simulink model "Cooperative_Localization_05"  (R2016b)
settings: Solver=ode45  StartTime=0.0  StopTime=300  RelTol=1e-3  EnableMultiTasking=on
InitFcn:
  | Const_Coop_Local_05
undefined symbols (not defined in the file): alpha, AN, B, B_pseudo_inverse, BBT_inv, BN, D, Delta_form, Gama0, gamma0, gamma_0, gamma_1, H, K, k0_est, k1, k1_est, k2, KI, Ki_1, Ki_2, Ki_3, Ki_4, lambda, m_cont, Mb, Mu, n, N, n_cont, Observer_Gain, P_struct, Q, Q1, R, Rho1, Rho_0, rho_0, rho_1, t_cont, U_dot0_M
(part 3 of 3)

== matlab function Cooperative_Localization_05/Agent-3/observer-1 ==
  data: P_hat input; tau input; P0 input; P_rel_local input; P_rel0_local input; AN parameter; BN parameter; H parameter; DP_hat_local output; n parameter; N parameter; Num input; Mu parameter; Mb parameter; tau_i output; alpha parameter
function [DP_hat_local,tau_i] = fcn(P_hat,tau,P0,P_rel_local,P_rel0_local,AN,BN,H,n,N,Num,Mu,Mb,alpha)

P_hat_in = zeros(n,N);
P_rel_local_in = zeros(n,N);
tau_in = zeros(n,N);
for i=1:N
    P_hat_in(:,i) = P_hat((i-1)*n+1:(i*n),1); 
    P_rel_local_in(:,i) = P_rel_local((i-1)*n+1:(i*n),1); 
    tau_in(:,i) = tau((i-1)*n+1:(i*n),1);
end

e = BN(Num,Num)*(P_hat_in(:,Num) - (P0 + P_rel0_local));
Vec = zeros(n,1);
for i=1:N
    e = e + ( AN(Num,i)*(P_hat_in(:,Num) - (P_hat_in(:,i) + P_rel_local_in(:,i))) ); 
    Vec = Vec + ( H(Num,i)*tau_in(:,i) );    
end

SGN_vec = Vec./(abs(Vec)+alpha);
SGN = diag(SGN_vec);    

DP_hat_local = - ( Mu*e ) - ( SGN*Mb );
tau_i = e;

end

== matlab function Cooperative_Localization_05/Agent-4/Agent-4/MATLAB Function ==
  data: Vx input; out output; Vy input; Ax input; Ay input
function out = fcn(Vx,Vy,Ax,Ay)

DPx = Vx;
DPy = Vy;

DVx = Ax;
DVy = Ay;

out = [DPx;DPy;DVx;DVy];

end

== matlab function Cooperative_Localization_05/Agent-4/Relative positions-4/Differentiator_Scalar1/Sliding differentiator ==
  data: u output; u1 input; e_inp input; k1 parameter
function u = fcn(u1,e_inp,k1)

b=k1;

if e_inp>0
    ABS = e_inp;
else
    ABS = -e_inp;
end

SGN = e_inp/(ABS + 0.01);

u = u1 - b*(ABS^0.5)*SGN;

end

== matlab function Cooperative_Localization_05/Agent-4/Relative positions-4/Differentiator_Scalar1/Sliding differentiator1 ==
  data: Du1 output; e_inp input; k2 parameter
function Du1 = fcn(e_inp,k2)

a=k2;

if e_inp>0
    ABS = e_inp;
else
    ABS = -e_inp;
end
SGN = e_inp/(ABS + 0.01);

Du1 = - a*SGN;

end

== matlab function Cooperative_Localization_05/Agent-4/Relative positions-4/Differentiator_Scalar2/Sliding differentiator ==
  data: u output; u1 input; e_inp input; k1 parameter
function u = fcn(u1,e_inp,k1)

b=k1;

if e_inp>0
    ABS = e_inp;
else
    ABS = -e_inp;
end

SGN = e_inp/(ABS + 0.01);

u = u1 - b*(ABS^0.5)*SGN;

end

== matlab function Cooperative_Localization_05/Agent-4/Relative positions-4/Differentiator_Scalar2/Sliding differentiator1 ==
  data: Du1 output; e_inp input; k2 parameter
function Du1 = fcn(e_inp,k2)

a=k2;

if e_inp>0
    ABS = e_inp;
else
    ABS = -e_inp;
end
SGN = e_inp/(ABS + 0.01);

Du1 = - a*SGN;

end

== matlab function Cooperative_Localization_05/Agent-4/Relative positions-4/Differentiator_Scalar3/Sliding differentiator ==
  data: u output; u1 input; e_inp input; k1 parameter
function u = fcn(u1,e_inp,k1)

b=k1;

if e_inp>0
    ABS = e_inp;
else
    ABS = -e_inp;
end

SGN = e_inp/(ABS + 0.01);

u = u1 - b*(ABS^0.5)*SGN;

end

== matlab function Cooperative_Localization_05/Agent-4/Relative positions-4/Differentiator_Scalar3/Sliding differentiator1 ==
  data: Du1 output; e_inp input; k2 parameter
function Du1 = fcn(e_inp,k2)

a=k2;

if e_inp>0
    ABS = e_inp;
else
    ABS = -e_inp;
end
SGN = e_inp/(ABS + 0.01);

Du1 = - a*SGN;

end

== matlab function Cooperative_Localization_05/Agent-4/Relative positions-4/Differentiator_Scalar4/Sliding differentiator ==
  data: u output; u1 input; e_inp input; k1 parameter
function u = fcn(u1,e_inp,k1)

b=k1;

if e_inp>0
    ABS = e_inp;
else
    ABS = -e_inp;
end

SGN = e_inp/(ABS + 0.01);

u = u1 - b*(ABS^0.5)*SGN;

end

== matlab function Cooperative_Localization_05/Agent-4/Relative positions-4/Differentiator_Scalar4/Sliding differentiator1 ==
  data: Du1 output; e_inp input; k2 parameter
function Du1 = fcn(e_inp,k2)

a=k2;

if e_inp>0
    ABS = e_inp;
else
    ABS = -e_inp;
end
SGN = e_inp/(ABS + 0.01);

Du1 = - a*SGN;

end

== matlab function Cooperative_Localization_05/Agent-4/Relative positions-4/Relative estimation1 ==
  data: V_rel input; d input; DP_est output; Dot_d input; P_est input; k0_est parameter; k1_est parameter
function DP_est = fcn(V_rel,d,Dot_d,P_est,k0_est,k1_est)

D = d*Dot_d;
e = (d^2) - (P_est'*P_est);
g = P_est'*V_rel;
DP_est = zeros(2,1);

if (V_rel'*V_rel) > 0
    beta = (k1_est*D + k0_est*e) / (k1_est*g+0.001);
    DP_est = beta * V_rel;
end

end

== matlab function Cooperative_Localization_05/Agent-4/Relative positions-4/Relative estimation2 ==
  data: V_rel input; d input; DP_est output; Dot_d input; P_est input; k0_est parameter; k1_est parameter
function DP_est = fcn(V_rel,d,Dot_d,P_est,k0_est,k1_est)

D = d*Dot_d;
e = (d^2) - (P_est'*P_est);
g = P_est'*V_rel;
DP_est = zeros(2,1);

if (V_rel'*V_rel) > 0
    beta = (k1_est*D + k0_est*e) / (k1_est*g+0.001);
    DP_est = beta * V_rel;
end

end

== matlab function Cooperative_Localization_05/Agent-4/Relative positions-4/Relative estimation3 ==
  data: V_rel input; d input; DP_est output; Dot_d input; P_est input; k0_est parameter; k1_est parameter
function DP_est = fcn(V_rel,d,Dot_d,P_est,k0_est,k1_est)

D = d*Dot_d;
e = (d^2) - (P_est'*P_est);
g = P_est'*V_rel;
DP_est = zeros(2,1);

if (V_rel'*V_rel) > 0
    beta = (k1_est*D + k0_est*e) / (k1_est*g+0.001);
    DP_est = beta * V_rel;
end

end

== matlab function Cooperative_Localization_05/Agent-4/Cooperative controller-4/Choosing real control variables ==
  data: u output; U input
function u = fcn(U)

u = U(3:4);

end

== matlab function Cooperative_Localization_05/Agent-4/Relative positions-4/Relative measurements ==
  data: P1 input; d output; P2 input
function d = fcn(P1,P2)

d = sqrt( (P2(1) - P1(1))^2 + (P2(2) - P1(2))^2 );

end

== matlab function Cooperative_Localization_05/Agent-4/Relative positions-4/Relative measurements1 ==
  data: P1 input; d output; P2 input
function d = fcn(P1,P2)

d = sqrt( (P2(1) - P1(1))^2 + (P2(2) - P1(2))^2 );

end

== matlab function Cooperative_Localization_05/Agent-4/Relative positions-4/Relative measurements2 ==
  data: P1 input; d output; P2 input
function d = fcn(P1,P2)

d = sqrt( (P2(1) - P1(1))^2 + (P2(2) - P1(2))^2 );

end

== matlab function Cooperative_Localization_05/Agent-4/Relative positions-4/Relative measurements3 ==
  data: P1 input; d output; P2 input
function d = fcn(P1,P2)

d = sqrt( (P2(1) - P1(1))^2 + (P2(2) - P1(2))^2 );

end

== matlab function Cooperative_Localization_05/Agent-4/Cooperative controller-4/Decenteralized Cooperaive Controller #4/Adaptive Law #4 ==
  data: Agent_Num input; G_hat input; Gama0 parameter; P input; P_struct parameter; DG_hat output; E input; H parameter; D parameter; N parameter; n_cont parameter; t_cont parameter; Rho_0 parameter
function DG_hat = fcn(Agent_Num,G_hat,Gama0,P,P_struct,E,H,D,N,n_cont,t_cont,Rho_0)

P_struct(1).data = P.p1;
P_struct(2).data = P.p2;
P_struct(3).data = P.p3;
P_struct(4).data = P.p4;

Sum = zeros(t_cont,1);
for i=1:N  
    Sum = Sum + (H(i,Agent_Num) * D' * P_struct(i).data * E((i-1)*n_cont+1:(i*n_cont),1)); %Adaptive law
end

DG_hat = +( Gama0*Sum - (Rho_0*Gama0*G_hat) );
    
end

== matlab function Cooperative_Localization_05/Agent-1/Cooperative controller-1/Decenteralized Cooperaive Controller #1/Approx. U#1 ==
  data: T_i input; Approx_U_i output; B_pseudo_inverse parameter; A_i input; X_i input; D parameter; G_hat_i input
function Approx_U_i  = fcn(T_i,B_pseudo_inverse,A_i,X_i,D,G_hat_i)

Approx_U_i = B_pseudo_inverse * (T_i - A_i * X_i + D * G_hat_i);

end

== matlab function Cooperative_Localization_05/Agent-4/observer-1 ==
  data: P_hat input; tau input; P0 input; P_rel_local input; P_rel0_local input; AN parameter; BN parameter; H parameter; DP_hat_local output; n parameter; N parameter; Num input; Mu parameter; Mb parameter; tau_i output; alpha parameter
function [DP_hat_local,tau_i] = fcn(P_hat,tau,P0,P_rel_local,P_rel0_local,AN,BN,H,n,N,Num,Mu,Mb,alpha)

P_hat_in = zeros(n,N);
P_rel_local_in = zeros(n,N);
tau_in = zeros(n,N);
for i=1:N
    P_hat_in(:,i) = P_hat((i-1)*n+1:(i*n),1); 
    P_rel_local_in(:,i) = P_rel_local((i-1)*n+1:(i*n),1); 
    tau_in(:,i) = tau((i-1)*n+1:(i*n),1);
end

e = BN(Num,Num)*(P_hat_in(:,Num) - (P0 + P_rel0_local));
Vec = zeros(n,1);
for i=1:N
    e = e + ( AN(Num,i)*(P_hat_in(:,Num) - (P_hat_in(:,i) + P_rel_local_in(:,i))) ); 
    Vec = Vec + ( H(Num,i)*tau_in(:,i) );    
end

SGN_vec = Vec./(abs(Vec)+alpha);
SGN = diag(SGN_vec);    

DP_hat_local = - ( Mu*e ) - ( SGN*Mb );
tau_i = e;

end

== matlab function Cooperative_Localization_05/Agent-1/Cooperative controller-1/Decenteralized Cooperaive Controller #1/Estimator A#1/For matrix Plot1/MATLAB Function ==
  data: u input; y output
function y = fcn(u)
S1 = size(u,1);
S2 = size(u,2);

y = zeros(S1*S2,1);
num = 0;
for i=1:S1
    for j=1:S2
        num = num + 1;
        y(num,1) = u(i,j);
    end
end

end

== matlab function Cooperative_Localization_05/Agent-1/Cooperative controller-1/Decenteralized Cooperaive Controller #1/Estimator A#1/For matrix Plot2/MATLAB Function ==
  data: u input; y output
function y = fcn(u)
S1 = size(u,1);
S2 = size(u,2);

y = zeros(S1*S2,1);
num = 0;
for i=1:S1
    for j=1:S2
        num = num + 1;
        y(num,1) = u(i,j);
    end
end

end

== matlab function Cooperative_Localization_05/Agent-1/Cooperative controller-1/Decenteralized Cooperaive Controller #1/Estimator A#1/parameter online identification ==
  data: r input; DA_hat output; Wt input; lambda parameter; A_hat input; Rho1 parameter; n_cont parameter
function DA_hat = fcn(r,Wt,lambda,A_hat,Rho1,n_cont)

eps = (Wt - A_hat*r)/(1+0.001);

DA_hat = (lambda * eps * r') - (Rho1 * lambda * A_hat); 

end

== matlab function Cooperative_Localization_05/Agent-1/Cooperative controller-1/Decenteralized Cooperaive Controller #1/For matrix Plot/MATLAB Function ==
  data: u input; y output
function y = fcn(u)
S1 = size(u,1);
S2 = size(u,2);

y = zeros(S1*S2,1);
num = 0;
for i=1:S1
    for j=1:S2
        num = num + 1;
        y(num,1) = u(i,j);
    end
end

end

== matlab function Cooperative_Localization_05/Agent-1/Cooperative controller-1/Decenteralized Cooperaive Controller #1/Main Controller #1 ==
  data: n_cont parameter; U output; K parameter; P_i input; E_i input; KI parameter; Zeta_i input; BN parameter; A_i input; U_0 input; Z_0 input; N parameter; H parameter; D parameter; B parameter; G_hat input; t_cont parameter; Delta_form parameter; m_cont parameter; Approx_U input; Agent_Num input; B_pseudo_inverse parameter
function U = fcn(n_cont,K,P_i,E_i,KI,Zeta_i,BN,A_i,U_0,Z_0,N,H,D,B,G_hat,t_cont,Delta_form,m_cont,Approx_U,Agent_Num,B_pseudo_inverse)

K_i = K((Agent_Num-1)*n_cont+1:(Agent_Num*n_cont),(Agent_Num-1)*n_cont+1:(Agent_Num*n_cont));
U1 = - K_i * P_i * E_i; %Consensus Error

KI_i = KI((Agent_Num-1)*n_cont+1:(Agent_Num*n_cont),(Agent_Num-1)*n_cont+1:(Agent_Num*n_cont));
U2 = - KI_i * Zeta_i; %Consensus time-integral

U3 = + BN(Agent_Num,Agent_Num)*(U_0-A_i*Z_0); %Connection to the leader

U4 = zeros(n_cont,1);
U5 = zeros(n_cont,1);
U6 = zeros(n_cont,1);
for i=1:N
    U4 = U4 - (H(Agent_Num,i)*A_i*Delta_form(:,i)); %Formation parameters
    
    U5 = U5 - (H(Agent_Num,i)*D*G_hat((i-1)*t_cont+1:(i*t_cont),1)); %Adaptive part
    
    if i~= Agent_Num
        U6 = U6 - (H(Agent_Num,i)*B*Approx_U((i-1)*m_cont+1:(i*m_cont),1)); %Observer on leader
    end
end

U_input = U1 + U2 + U3 + U4 + U5 + U6;

U = B_pseudo_inverse * U_input / H(Agent_Num,Agent_Num);

end

== matlab function Cooperative_Localization_05/Agent-1/Cooperative controller-1/Decenteralized Cooperaive Controller #1/Observer #1 ==
  data: T input; DT_i output; Delta input; H parameter; BN parameter; AN parameter; T_i input; U0 input; U_dot0_M parameter; Delta_i output; N parameter; n_cont parameter; Agent_Num input; Observer_Gain parameter
function [DT_i,Delta_i] = fcn(T,Delta,H,BN,AN,T_i,U0,U_dot0_M,N,n_cont,Agent_Num,Observer_Gain)

Delta_i = + BN(Agent_Num,Agent_Num)*(T_i - U0);
Sum2 = zeros(n_cont,1);
for i=1:N
    Delta_i = Delta_i + ( AN(Agent_Num,i) * (T_i - T(((i-1)*n_cont+1):n_cont*i)) );  
    Sum2 = Sum2 + ( H(i,Agent_Num) * Delta(((i-1)*n_cont+1):n_cont*i) );
end

Sum21 = abs(Sum2) + 0.01*ones(n_cont,1);
SGN2 = Sum2./Sum21;

DT_i = -Observer_Gain*Delta_i - diag(SGN2)*U_dot0_M;

end

== matlab function Cooperative_Localization_05/Agent-1/Cooperative controller-1/Decenteralized Cooperaive Controller #1/Riccati equation ==
  data: A_hat input; K_i input; Q parameter; P_i output; gamma0 parameter; n_cont parameter
function P_i = care_sol(A_hat,K_i,Q,gamma0,n_cont)

% Reference: "Numerical Solution of Algebraic Riccati Equations" by: "Dario A. Bini" - Page 194 in PDF.
% CARE: A'X + XA - XBX = -C
% gamma should be negative EX. = -1;

A = A_hat + 1e-3*eye(n_cont);
B = K_i;
C = Q;
gamma = gamma0;

tol = 1e-13;
kmax = 30;

Ai = inv(A+(gamma*eye(n_cont)));
R = B*Ai'*C;
S1 = inv(A+(gamma*eye(n_cont))+R);
E = S1*(A-(gamma*eye(n_cont))+R);
R = eye(n_cont)-(Ai*(A-(gamma*eye(n_cont))));
G = S1*B*R';
P = -S1'*C*R;

err = 1;
ki = 0;

while err>tol && ki<kmax
    IGP = eye(n_cont) - G*P;
    Z = [E;P']/IGP;
    E1 = Z(1:n_cont,:);
    P1 = Z(n_cont+1:end,:);
    G = G + (E1*G*E');
    P = P + (E'*P1'*E);
    E = E1*E;
    err = norm(E,1);
    ki = ki+1;
end

P_i = P;

end

== matlab function Cooperative_Localization_05/Agent-1/Cooperative controller-1/Module to compute Consensus Error #1 ==
  data: P_rel_all input; P_rel0 input; V_loc input; V0 input; V_all input; Ep output; AN parameter; BN parameter; Delta_form parameter; N parameter; n_cont parameter; Agent_Num input; n parameter
function Ep = fcn(P_rel_all,P_rel0,V_loc,V0,V_all,AN,BN,Delta_form,N,n_cont,Agent_Num, n)

Diff_Star_to0 = Delta_form(:,Agent_Num); 
Diff_Star_to_Other = ( eye(n_cont) * Diff_Star_to0 * ones(1,N) ) - Delta_form;

%% ---------------------------------------------------------------

Ep = ( BN(Agent_Num,Agent_Num)*([P_rel0;(V_loc-V0)]-Diff_Star_to0) ); 

for i=1:N        
    Ep = Ep + AN(Agent_Num,i)*([P_rel_all((n*(i-1)+1):(i*n),1);(V_loc-V_all((n*(i-1)+1):(i*n),1))]-Diff_Star_to_Other(:,i));
end

end

== matlab function Cooperative_Localization_05/Agent-1/Cooperative controller-1/Variable change ==
  data: U input; X input; X_mod output; n_cont parameter
function X_mod = fcn(U,X,n_cont)

X_mod = zeros(n_cont,1);
X_mod(1:2) = X(1:2);
X_mod(3:4) = X(3:4) - U(1:2);

end

== matlab function Cooperative_Localization_05/Agent-2/Cooperative controller-2/Module to compute Consensus Error #2 ==
  data: P_rel_all input; P_rel0 input; V_loc input; V0 input; V_all input; Ep output; AN parameter; BN parameter; Delta_form parameter; N parameter; n_cont parameter; Agent_Num input; n parameter
function Ep = fcn(P_rel_all,P_rel0,V_loc,V0,V_all,AN,BN,Delta_form,N,n_cont,Agent_Num, n)

Diff_Star_to0 = Delta_form(:,Agent_Num); 
Diff_Star_to_Other = ( eye(n_cont) * Diff_Star_to0 * ones(1,N) ) - Delta_form;

%% ---------------------------------------------------------------

Ep = ( BN(Agent_Num,Agent_Num)*([P_rel0;(V_loc-V0)]-Diff_Star_to0) );

for i=1:N        
    Ep = Ep + AN(Agent_Num,i)*([P_rel_all((n*(i-1)+1):(i*n),1);(V_loc-V_all((n*(i-1)+1):(i*n),1))]-Diff_Star_to_Other(:,i));
end

end

== matlab function Cooperative_Localization_05/Agent-2/Cooperative controller-2/Decenteralized Cooperaive Controller #2/Approx. U#2 ==
  data: T_i input; Approx_U_i output; B_pseudo_inverse parameter; A_i input; X_i input; D parameter; G_hat_i input
function Approx_U_i  = fcn(T_i,B_pseudo_inverse,A_i,X_i,D,G_hat_i)

Approx_U_i = B_pseudo_inverse * (T_i - A_i * X_i + D * G_hat_i);

end

== matlab function Cooperative_Localization_05/Agent-2/Cooperative controller-2/Decenteralized Cooperaive Controller #2/Estimator A#2/For matrix Plot1/MATLAB Function ==
  data: u input; y output
function y = fcn(u)
S1 = size(u,1);
S2 = size(u,2);

y = zeros(S1*S2,1);
num = 0;
for i=1:S1
    for j=1:S2
        num = num + 1;
        y(num,1) = u(i,j);
    end
end

end

== matlab function Cooperative_Localization_05/Agent-2/Cooperative controller-2/Decenteralized Cooperaive Controller #2/Estimator A#2/For matrix Plot2/MATLAB Function ==
  data: u input; y output
function y = fcn(u)
S1 = size(u,1);
S2 = size(u,2);

y = zeros(S1*S2,1);
num = 0;
for i=1:S1
    for j=1:S2
        num = num + 1;
        y(num,1) = u(i,j);
    end
end

end

== matlab function Cooperative_Localization_05/Agent-2/Cooperative controller-2/Decenteralized Cooperaive Controller #2/Estimator A#2/parameter online identification ==
  data: r input; DA_hat output; Wt input; lambda parameter; A_hat input; Rho1 parameter; n_cont parameter
function DA_hat = fcn(r,Wt,lambda,A_hat,Rho1,n_cont)

eps = (Wt - A_hat*r)/(1+0.001);

DA_hat = (lambda * eps * r') - (Rho1 * lambda * A_hat); 

end

== matlab function Cooperative_Localization_05/Agent-2/Cooperative controller-2/Decenteralized Cooperaive Controller #2/For matrix Plot/MATLAB Function ==
  data: u input; y output
function y = fcn(u)
S1 = size(u,1);
S2 = size(u,2);

y = zeros(S1*S2,1);
num = 0;
for i=1:S1
    for j=1:S2
        num = num + 1;
        y(num,1) = u(i,j);
    end
end

end

== matlab function Cooperative_Localization_05/Agent-2/Cooperative controller-2/Decenteralized Cooperaive Controller #2/Main Controller #2 ==
  data: n_cont parameter; U output; K parameter; P_i input; E_i input; KI parameter; Zeta_i input; BN parameter; A_i input; U_0 input; Z_0 input; N parameter; H parameter; D parameter; B parameter; G_hat input; t_cont parameter; Delta_form parameter; m_cont parameter; Approx_U input; Agent_Num input; B_pseudo_inverse parameter
function U = fcn(n_cont,K,P_i,E_i,KI,Zeta_i,BN,A_i,U_0,Z_0,N,H,D,B,G_hat,t_cont,Delta_form,m_cont,Approx_U,Agent_Num,B_pseudo_inverse)

K_i = K((Agent_Num-1)*n_cont+1:(Agent_Num*n_cont),(Agent_Num-1)*n_cont+1:(Agent_Num*n_cont));
U1 = - K_i * P_i * E_i; %Consensus Error

KI_i = KI((Agent_Num-1)*n_cont+1:(Agent_Num*n_cont),(Agent_Num-1)*n_cont+1:(Agent_Num*n_cont));
U2 = - KI_i * Zeta_i; %Consensus time-integral

U3 = + BN(Agent_Num,Agent_Num)*(U_0-A_i*Z_0); %Connection to the leader

U4 = zeros(n_cont,1);
U5 = zeros(n_cont,1);
U6 = zeros(n_cont,1);
for i=1:N
    U4 = U4 - (H(Agent_Num,i)*A_i*Delta_form(:,i)); %Formation parameters
    
    U5 = U5 - (H(Agent_Num,i)*D*G_hat((i-1)*t_cont+1:(i*t_cont),1)); %Adaptive part
    
    if i~= Agent_Num
        U6 = U6 - (H(Agent_Num,i)*B*Approx_U((i-1)*m_cont+1:(i*m_cont),1)); %Observer on leader
    end
end

U_input = U1 + U2 + U3 + U4 + U5 + U6;

U = B_pseudo_inverse * U_input / H(Agent_Num,Agent_Num);

end

== matlab function Cooperative_Localization_05/Agent-2/Cooperative controller-2/Decenteralized Cooperaive Controller #2/Observer #2 ==
  data: T input; DT_i output; Delta input; H parameter; BN parameter; AN parameter; T_i input; U0 input; U_dot0_M parameter; Delta_i output; N parameter; n_cont parameter; Agent_Num input; Observer_Gain parameter
function [DT_i,Delta_i] = fcn(T,Delta,H,BN,AN,T_i,U0,U_dot0_M,N,n_cont,Agent_Num,Observer_Gain)

Delta_i = + BN(Agent_Num,Agent_Num)*(T_i - U0);
Sum2 = zeros(n_cont,1);
for i=1:N
    Delta_i = Delta_i + ( AN(Agent_Num,i) * (T_i - T(((i-1)*n_cont+1):n_cont*i)) );  
    Sum2 = Sum2 + ( H(i,Agent_Num) * Delta(((i-1)*n_cont+1):n_cont*i) );
end

Sum21 = abs(Sum2) + 0.01*ones(n_cont,1);
SGN2 = Sum2./Sum21;

DT_i = -Observer_Gain*Delta_i - diag(SGN2)*U_dot0_M;

end

== matlab function Cooperative_Localization_05/Agent-2/Cooperative controller-2/Decenteralized Cooperaive Controller #2/Riccati equation ==
  data: A_hat input; K_i input; Q parameter; P_i output; gamma0 parameter; n_cont parameter
function P_i = care_sol(A_hat,K_i,Q,gamma0,n_cont)

% Reference: "Numerical Solution of Algebraic Riccati Equations" by: "Dario A. Bini" - Page 194 in PDF.
% CARE: A'X + XA - XBX = -C
% gamma should be negative EX. = -1;

A = A_hat + 1e-3*eye(n_cont);
B = K_i;
C = Q;
gamma = gamma0;

tol = 1e-13;
kmax = 30;

Ai = inv(A+(gamma*eye(n_cont)));
R = B*Ai'*C;
S1 = inv(A+(gamma*eye(n_cont))+R);
E = S1*(A-(gamma*eye(n_cont))+R);
R = eye(n_cont)-(Ai*(A-(gamma*eye(n_cont))));
G = S1*B*R';
P = -S1'*C*R;

err = 1;
ki = 0;

while err>tol && ki<kmax
    IGP = eye(n_cont) - G*P;
    Z = [E;P']/IGP;
    E1 = Z(1:n_cont,:);
    P1 = Z(n_cont+1:end,:);
    G = G + (E1*G*E');
    P = P + (E'*P1'*E);
    E = E1*E;
    err = norm(E,1);
    ki = ki+1;
end

P_i = P;

end

== matlab function Cooperative_Localization_05/Agent-3/Cooperative controller-3/Module to compute Consensus Error #3 ==
  data: P_rel_all input; P_rel0 input; V_loc input; V0 input; V_all input; Ep output; AN parameter; BN parameter; Delta_form parameter; N parameter; n_cont parameter; Agent_Num input; n parameter
function Ep = fcn(P_rel_all,P_rel0,V_loc,V0,V_all,AN,BN,Delta_form,N,n_cont,Agent_Num, n)

Diff_Star_to0 = Delta_form(:,Agent_Num); 
Diff_Star_to_Other = ( eye(n_cont) * Diff_Star_to0 * ones(1,N) ) - Delta_form;

%% ---------------------------------------------------------------

Ep = ( BN(Agent_Num,Agent_Num)*([P_rel0;(V_loc-V0)]-Diff_Star_to0) );

for i=1:N        
    Ep = Ep + AN(Agent_Num,i)*([P_rel_all((n*(i-1)+1):(i*n),1);(V_loc-V_all((n*(i-1)+1):(i*n),1))]-Diff_Star_to_Other(:,i));
end

end

== matlab function Cooperative_Localization_05/Agent-2/Cooperative controller-2/Variable change ==
  data: U input; X input; X_mod output; n_cont parameter
function X_mod = fcn(U,X,n_cont)

X_mod = zeros(n_cont,1);
X_mod(1:2) = X(1:2);
X_mod(3:4) = X(3:4) - U(1:2);

end

== matlab function Cooperative_Localization_05/Agent-3/Cooperative controller-3/Decenteralized Cooperaive Controller #3/Approx. U#3 ==
  data: T_i input; Approx_U_i output; B_pseudo_inverse parameter; A_i input; X_i input; D parameter; G_hat_i input
function Approx_U_i  = fcn(T_i,B_pseudo_inverse,A_i,X_i,D,G_hat_i)

Approx_U_i = B_pseudo_inverse * (T_i - A_i * X_i + D * G_hat_i);

end

== matlab function Cooperative_Localization_05/Agent-3/Cooperative controller-3/Decenteralized Cooperaive Controller #3/Estimator A#3/For matrix Plot1/MATLAB Function ==
  data: u input; y output
function y = fcn(u)
S1 = size(u,1);
S2 = size(u,2);

y = zeros(S1*S2,1);
num = 0;
for i=1:S1
    for j=1:S2
        num = num + 1;
        y(num,1) = u(i,j);
    end
end

end

== matlab function Cooperative_Localization_05/Agent-3/Cooperative controller-3/Decenteralized Cooperaive Controller #3/Estimator A#3/For matrix Plot2/MATLAB Function ==
  data: u input; y output
function y = fcn(u)
S1 = size(u,1);
S2 = size(u,2);

y = zeros(S1*S2,1);
num = 0;
for i=1:S1
    for j=1:S2
        num = num + 1;
        y(num,1) = u(i,j);
    end
end

end

== matlab function Cooperative_Localization_05/Agent-3/Cooperative controller-3/Decenteralized Cooperaive Controller #3/Estimator A#3/parameter online identification ==
  data: r input; DA_hat output; Wt input; lambda parameter; A_hat input; Rho1 parameter; n_cont parameter
function DA_hat = fcn(r,Wt,lambda,A_hat,Rho1,n_cont)

eps = (Wt - A_hat*r)/(1+0.001);

DA_hat = (lambda * eps * r') - (Rho1 * lambda * A_hat); 

end

== matlab function Cooperative_Localization_05/Agent-3/Cooperative controller-3/Decenteralized Cooperaive Controller #3/For matrix Plot/MATLAB Function ==
  data: u input; y output
function y = fcn(u)
S1 = size(u,1);
S2 = size(u,2);

y = zeros(S1*S2,1);
num = 0;
for i=1:S1
    for j=1:S2
        num = num + 1;
        y(num,1) = u(i,j);
    end
end

end

== matlab function Cooperative_Localization_05/Agent-3/Cooperative controller-3/Decenteralized Cooperaive Controller #3/Main Controller #3 ==
  data: n_cont parameter; U output; K parameter; P_i input; E_i input; KI parameter; Zeta_i input; BN parameter; A_i input; U_0 input; Z_0 input; N parameter; H parameter; D parameter; B parameter; G_hat input; t_cont parameter; Delta_form parameter; m_cont parameter; Approx_U input; Agent_Num input; B_pseudo_inverse parameter
function U = fcn(n_cont,K,P_i,E_i,KI,Zeta_i,BN,A_i,U_0,Z_0,N,H,D,B,G_hat,t_cont,Delta_form,m_cont,Approx_U,Agent_Num,B_pseudo_inverse)

K_i = K((Agent_Num-1)*n_cont+1:(Agent_Num*n_cont),(Agent_Num-1)*n_cont+1:(Agent_Num*n_cont));
U1 = - K_i * P_i * E_i; %Consensus Error

KI_i = KI((Agent_Num-1)*n_cont+1:(Agent_Num*n_cont),(Agent_Num-1)*n_cont+1:(Agent_Num*n_cont));
U2 = - KI_i * Zeta_i; %Consensus time-integral

U3 = + BN(Agent_Num,Agent_Num)*(U_0-A_i*Z_0); %Connection to the leader

U4 = zeros(n_cont,1);
U5 = zeros(n_cont,1);
U6 = zeros(n_cont,1);
for i=1:N
    U4 = U4 - (H(Agent_Num,i)*A_i*Delta_form(:,i)); %Formation parameters
    
    U5 = U5 - (H(Agent_Num,i)*D*G_hat((i-1)*t_cont+1:(i*t_cont),1)); %Adaptive part
    
    if i~= Agent_Num
        U6 = U6 - (H(Agent_Num,i)*B*Approx_U((i-1)*m_cont+1:(i*m_cont),1)); %Observer on leader
    end
end

U_input = U1 + U2 + U3 + U4 + U5 + U6;

U = B_pseudo_inverse * U_input / H(Agent_Num,Agent_Num);

end

== matlab function Cooperative_Localization_05/Agent-3/Cooperative controller-3/Decenteralized Cooperaive Controller #3/Observer #3 ==
  data: T input; DT_i output; Delta input; H parameter; BN parameter; AN parameter; T_i input; U0 input; U_dot0_M parameter; Delta_i output; N parameter; n_cont parameter; Agent_Num input; Observer_Gain parameter
function [DT_i,Delta_i] = fcn(T,Delta,H,BN,AN,T_i,U0,U_dot0_M,N,n_cont,Agent_Num,Observer_Gain)

Delta_i = + BN(Agent_Num,Agent_Num)*(T_i - U0);
Sum2 = zeros(n_cont,1);
for i=1:N
    Delta_i = Delta_i + ( AN(Agent_Num,i) * (T_i - T(((i-1)*n_cont+1):n_cont*i)) );  
    Sum2 = Sum2 + ( H(i,Agent_Num) * Delta(((i-1)*n_cont+1):n_cont*i) );
end

Sum21 = abs(Sum2) + 0.01*ones(n_cont,1);
SGN2 = Sum2./Sum21;

DT_i = -Observer_Gain*Delta_i - diag(SGN2)*U_dot0_M;

end

== matlab function Cooperative_Localization_05/Agent-3/Cooperative controller-3/Decenteralized Cooperaive Controller #3/Riccati equation ==
  data: A_hat input; K_i input; Q parameter; P_i output; gamma0 parameter; n_cont parameter
function P_i = care_sol(A_hat,K_i,Q,gamma0,n_cont)

% Reference: "Numerical Solution of Algebraic Riccati Equations" by: "Dario A. Bini" - Page 194 in PDF.
% CARE: A'X + XA - XBX = -C
% gamma should be negative EX. = -1;

A = A_hat + 1e-3*eye(n_cont);
B = K_i;
C = Q;
gamma = gamma0;

tol = 1e-13;
kmax = 30;

Ai = inv(A+(gamma*eye(n_cont)));
R = B*Ai'*C;
S1 = inv(A+(gamma*eye(n_cont))+R);
E = S1*(A-(gamma*eye(n_cont))+R);
R = eye(n_cont)-(Ai*(A-(gamma*eye(n_cont))));
G = S1*B*R';
P = -S1'*C*R;

err = 1;
ki = 0;

while err>tol && ki<kmax
    IGP = eye(n_cont) - G*P;
    Z = [E;P']/IGP;
    E1 = Z(1:n_cont,:);
    P1 = Z(n_cont+1:end,:);
    G = G + (E1*G*E');
    P = P + (E'*P1'*E);
    E = E1*E;
    err = norm(E,1);
    ki = ki+1;
end

P_i = P;

end

== matlab function Cooperative_Localization_05/Agent-4/Cooperative controller-4/Module to compute Consensus Error #4 ==
  data: P_rel_all input; P_rel0 input; V_loc input; V0 input; V_all input; Ep output; AN parameter; BN parameter; Delta_form parameter; N parameter; n_cont parameter; Agent_Num input; n parameter
function Ep = fcn(P_rel_all,P_rel0,V_loc,V0,V_all,AN,BN,Delta_form,N,n_cont,Agent_Num, n)

Diff_Star_to0 = Delta_form(:,Agent_Num); 
Diff_Star_to_Other = ( eye(n_cont) * Diff_Star_to0 * ones(1,N) ) - Delta_form;

%% ---------------------------------------------------------------

Ep = ( BN(Agent_Num,Agent_Num)*([P_rel0;(V_loc-V0)]-Diff_Star_to0) );

for i=1:N        
    Ep = Ep + AN(Agent_Num,i)*([P_rel_all((n*(i-1)+1):(i*n),1);(V_loc-V_all((n*(i-1)+1):(i*n),1))]-Diff_Star_to_Other(:,i));
end

end

== matlab function Cooperative_Localization_05/Agent-3/Cooperative controller-3/Variable change ==
  data: U input; X input; X_mod output; n_cont parameter
function X_mod = fcn(U,X,n_cont)

X_mod = zeros(n_cont,1);
X_mod(1:2) = X(1:2);
X_mod(3:4) = X(3:4) - U(1:2);

end

== matlab function Cooperative_Localization_05/Agent-4/Cooperative controller-4/Decenteralized Cooperaive Controller #4/Approx. U#4 ==
  data: T_i input; Approx_U_i output; B_pseudo_inverse parameter; A_i input; X_i input; D parameter; G_hat_i input
function Approx_U_i  = fcn(T_i,B_pseudo_inverse,A_i,X_i,D,G_hat_i)

Approx_U_i = B_pseudo_inverse * (T_i - A_i * X_i + D * G_hat_i);

end

== matlab function Cooperative_Localization_05/Agent-4/Cooperative controller-4/Decenteralized Cooperaive Controller #4/Estimator A#4/For matrix Plot1/MATLAB Function ==
  data: u input; y output
function y = fcn(u)
S1 = size(u,1);
S2 = size(u,2);

y = zeros(S1*S2,1);
num = 0;
for i=1:S1
    for j=1:S2
        num = num + 1;
        y(num,1) = u(i,j);
    end
end

end

== matlab function Cooperative_Localization_05/Agent-4/Cooperative controller-4/Decenteralized Cooperaive Controller #4/Estimator A#4/For matrix Plot2/MATLAB Function ==
  data: u input; y output
function y = fcn(u)
S1 = size(u,1);
S2 = size(u,2);

y = zeros(S1*S2,1);
num = 0;
for i=1:S1
    for j=1:S2
        num = num + 1;
        y(num,1) = u(i,j);
    end
end

end

== matlab function Cooperative_Localization_05/Agent-4/Cooperative controller-4/Decenteralized Cooperaive Controller #4/Estimator A#4/parameter online identification ==
  data: r input; DA_hat output; Wt input; lambda parameter; A_hat input; Rho1 parameter; n_cont parameter
function DA_hat = fcn(r,Wt,lambda,A_hat,Rho1,n_cont)

eps = (Wt - A_hat*r)/(1+0.001);

DA_hat = (lambda * eps * r') - (Rho1 * lambda * A_hat); 

end

== matlab function Cooperative_Localization_05/Agent-4/Cooperative controller-4/Decenteralized Cooperaive Controller #4/For matrix Plot/MATLAB Function ==
  data: u input; y output
function y = fcn(u)
S1 = size(u,1);
S2 = size(u,2);

y = zeros(S1*S2,1);
num = 0;
for i=1:S1
    for j=1:S2
        num = num + 1;
        y(num,1) = u(i,j);
    end
end

end

== matlab function Cooperative_Localization_05/Agent-4/Cooperative controller-4/Decenteralized Cooperaive Controller #4/Main Controller #4 ==
  data: n_cont parameter; U output; K parameter; P_i input; E_i input; KI parameter; Zeta_i input; BN parameter; A_i input; U_0 input; Z_0 input; N parameter; H parameter; D parameter; B parameter; G_hat input; t_cont parameter; Delta_form parameter; m_cont parameter; Approx_U input; Agent_Num input; B_pseudo_inverse parameter
function U = fcn(n_cont,K,P_i,E_i,KI,Zeta_i,BN,A_i,U_0,Z_0,N,H,D,B,G_hat,t_cont,Delta_form,m_cont,Approx_U,Agent_Num,B_pseudo_inverse)

K_i = K((Agent_Num-1)*n_cont+1:(Agent_Num*n_cont),(Agent_Num-1)*n_cont+1:(Agent_Num*n_cont));
U1 = - K_i * P_i * E_i; %Consensus Error

KI_i = KI((Agent_Num-1)*n_cont+1:(Agent_Num*n_cont),(Agent_Num-1)*n_cont+1:(Agent_Num*n_cont));
U2 = - KI_i * Zeta_i; %Consensus time-integral

U3 = + BN(Agent_Num,Agent_Num)*(U_0-A_i*Z_0); %Connection to the leader

U4 = zeros(n_cont,1);
U5 = zeros(n_cont,1);
U6 = zeros(n_cont,1);
for i=1:N
    U4 = U4 - (H(Agent_Num,i)*A_i*Delta_form(:,i)); %Formation parameters
    
    U5 = U5 - (H(Agent_Num,i)*D*G_hat((i-1)*t_cont+1:(i*t_cont),1)); %Adaptive part
    
    if i~= Agent_Num
        U6 = U6 - (H(Agent_Num,i)*B*Approx_U((i-1)*m_cont+1:(i*m_cont),1)); %Observer on leader
    end
end

U_input = U1 + U2 + U3 + U4 + U5 + U6;

U = B_pseudo_inverse * U_input / H(Agent_Num,Agent_Num);

end

== matlab function Cooperative_Localization_05/Agent-4/Cooperative controller-4/Decenteralized Cooperaive Controller #4/Observer #4 ==
  data: T input; DT_i output; Delta input; H parameter; BN parameter; AN parameter; T_i input; U0 input; U_dot0_M parameter; Delta_i output; N parameter; n_cont parameter; Agent_Num input; Observer_Gain parameter
function [DT_i,Delta_i] = fcn(T,Delta,H,BN,AN,T_i,U0,U_dot0_M,N,n_cont,Agent_Num,Observer_Gain)

Delta_i = + BN(Agent_Num,Agent_Num)*(T_i - U0);
Sum2 = zeros(n_cont,1);
for i=1:N
    Delta_i = Delta_i + ( AN(Agent_Num,i) * (T_i - T(((i-1)*n_cont+1):n_cont*i)) );  
    Sum2 = Sum2 + ( H(i,Agent_Num) * Delta(((i-1)*n_cont+1):n_cont*i) );
end

Sum21 = abs(Sum2) + 0.01*ones(n_cont,1);
SGN2 = Sum2./Sum21;

DT_i = -Observer_Gain*Delta_i - diag(SGN2)*U_dot0_M;

end

== matlab function Cooperative_Localization_05/Agent-4/Cooperative controller-4/Decenteralized Cooperaive Controller #4/Riccati equation ==
  data: A_hat input; K_i input; Q parameter; P_i output; gamma0 parameter; n_cont parameter
function P_i = care_sol(A_hat,K_i,Q,gamma0,n_cont)

% Reference: "Numerical Solution of Algebraic Riccati Equations" by: "Dario A. Bini" - Page 194 in PDF.
% CARE: A'X + XA - XBX = -C
% gamma should be negative EX. = -1;

A = A_hat + 1e-3*eye(n_cont);
B = K_i;
C = Q;
gamma = gamma0;

tol = 1e-13;
kmax = 30;

Ai = inv(A+(gamma*eye(n_cont)));
R = B*Ai'*C;
S1 = inv(A+(gamma*eye(n_cont))+R);
E = S1*(A-(gamma*eye(n_cont))+R);
R = eye(n_cont)-(Ai*(A-(gamma*eye(n_cont))));
G = S1*B*R';
P = -S1'*C*R;

err = 1;
ki = 0;

while err>tol && ki<kmax
    IGP = eye(n_cont) - G*P;
    Z = [E;P']/IGP;
    E1 = Z(1:n_cont,:);
    P1 = Z(n_cont+1:end,:);
    G = G + (E1*G*E');
    P = P + (E'*P1'*E);
    E = E1*E;
    err = norm(E,1);
    ki = ki+1;
end

P_i = P;

end

== matlab function Cooperative_Localization_05/Leader/Agent-0/MATLAB Function ==
  data: Vx input; out output; Vy input; Ax input; Ay input
function out = fcn(Vx,Vy,Ax,Ay)

DPx = Vx;
DPy = Vy;

DVx = Ax;
DVy = Ay;

out = [DPx;DPy;DVx;DVy];

end

== matlab function Cooperative_Localization_05/Agent-4/Cooperative controller-4/Variable change ==
  data: U input; X input; X_mod output; n_cont parameter
function X_mod = fcn(U,X,n_cont)

X_mod = zeros(n_cont,1);
X_mod(1:2) = X(1:2);
X_mod(3:4) = X(3:4) - U(1:2);

end

== matlab function Cooperative_Localization_05/Leader/Ali/CARE ==
  data: P input; a_hat input; B parameter; R parameter; DP output; Q1 parameter
function DP = fcn(P,a_hat,B,R,Q1)

DP = a_hat*P + P*a_hat' - P*B*R*B'*P + 2*Q1;

end

== matlab function Cooperative_Localization_05/Leader/Ali/Differentiator/Sliding differentiator ==
  data: u output; u1 input; e input; n_cont parameter; k1 parameter
function u = fcn(u1,e,n_cont,k1)

b=k1;

ABS = zeros(n_cont,1);
for i=1:n_cont
    if e(i)>0
        ABS(i) = e(i);
    else
        ABS(i) = -e(i);
    end
end
SGN = e ./ (ABS + 0.01);

u = u1 - b*(ABS.^0.5).*SGN;

end

== matlab function Cooperative_Localization_05/Leader/Ali/Differentiator/Sliding differentiator1 ==
  data: Du1 output; e input; n_cont parameter; k2 parameter
function Du1 = fcn(e,n_cont,k2)

a=k2;

ABS = zeros(n_cont,1);
for i=1:n_cont
    if e(i)>0
        ABS(i) = e(i);
    else
        ABS(i) = -e(i);
    end
end
SGN = e ./ (ABS + 0.01);

Du1 = - a*SGN;

end

== matlab function Cooperative_Localization_05/Leader/Ali/g-Estimator ==
  data: sigma input; g_hat input; P input; rho_1 parameter; gamma_1 parameter; Dg_hat output
function Dg_hat = fcn(sigma,g_hat,P,rho_1,gamma_1)

Dg_hat = - gamma_1 * P * sigma - rho_1 * gamma_1 * g_hat;

end

== matlab function Cooperative_Localization_05/Leader/Ali/g-Estimator1 ==
  data: sigma input; x input; P input; rho_0 parameter; gamma_0 parameter; Da_hat output; a_hat input
function Da_hat = fcn(sigma,x,P,rho_0,gamma_0,a_hat)

DVa_hat = - gamma_0 * P * diag(sigma) * (x - sigma) - rho_0 * gamma_0 * diag(a_hat);

Da_hat = diag(DVa_hat);

end

== matlab function Cooperative_Localization_05/Leader/Ali/main ==
  data: sigma input; zeta input; u output; Dy_d input; R parameter; P input; a_hat input; B parameter; g_hat input; x input; Q1 parameter; BBT_inv parameter; n_cont parameter
function u = fcn(sigma,zeta,Dy_d,R,P,a_hat,B,g_hat,x,Q1,BBT_inv,n_cont)

u = zeros(n_cont,1);

u1 = (1/2) * R * B' * P * sigma;
u2 = BBT_inv * (Dy_d - a_hat*x + (eye(n_cont) + 2*(((P)^(-1)*Q1)) + a_hat)*sigma - g_hat - zeta) - (3/4) * R * B' * P * sigma;

u(1:4,1) = u1 + u2;

end

== matlab function Cooperative_Localization_05/Leader/Ali/variable change ==
  data: X input; Xd input; x_mod output; u input; xd_mod output; e_mod output
function [x_mod,xd_mod,e_mod] = fcn(X,Xd,u)

x_mod = X(1:4);

xd_mod = [Xd;u(1:2)];

e_mod = xd_mod - x_mod;


end

== matlab function Cooperative_Localization_05/Leader/Controller interpreter ==
  data: u output; U input
function u = fcn(U)

u = U(3:4);

end
